simulink model "Switch"  (R2017b)
settings: Solver=FixedStepAuto  StartTime=0.0  StopTime=10.0  FixedStep=0.1  RelTol=1e-3  EnableMultiTasking=on
settings Model: Creator=ktrinh  LastModifiedBy=hbourbou
settings DataIOCC: SaveFormat=StructureWithTime
settings OptimizationCC: LifeSpan=inf
settings DebuggingCC: SFUnexpectedBacktrackingDiag=warning  SFNoUnconditionalDefaultTransitionDiag=warning  SFExecutionAtInitializationDiag=none
settings HardwareCC: ProdBitPerSizeT=32  ProdBitPerPtrDiffT=32  ProdWordSize=32  ProdHWDeviceType=Specified
settings CodeAppCC: StateflowObjectComments=on
settings GRTTargetCC: TargetLangStandard=C89/C90 (ANSI)  GeneratePreprocessorConditionals=Disable all
settings ConfigComp: CovMetricSettings=dw  CovHtmlReporting=on  CovSaveCumulativeToWorkspaceVar=on  CovSaveSingleToWorkspaceVar=on  CovExternalEMLEnable=off

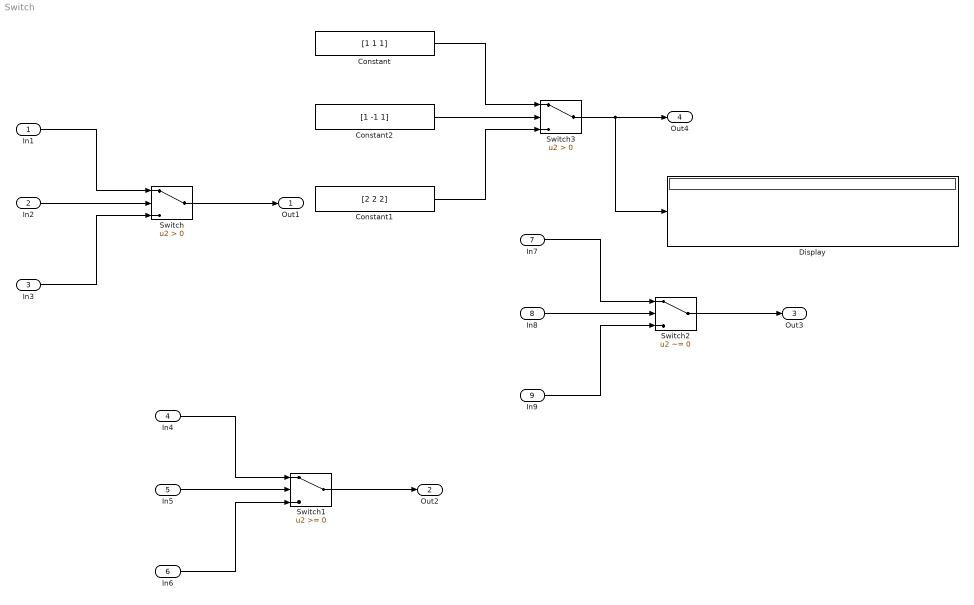
== system Switch ==
  In1 : Inport  OutMin=5  OutDataTypeStr=uint8  PortDimensions=3
  In2 : Inport  Port=2  PortDimensions=3
  In3 : Inport  Port=3  PortDimensions=3
  In4 : Inport  Port=4
  In5 : Inport  Port=5
  In6 : Inport  Port=6
  In7 : Inport  Port=7
  In8 : Inport  Port=8
  In9 : Inport  Port=9
  Constant : Constant  Value=[1 1 1]
  Constant1 : Constant  Value=[2 2 2]
  Constant2 : Constant  Value=[1 -1 1]
  Display : Display
  Switch : Switch  Criteria=u2 > Threshold
  Switch1 : Switch
  Switch2 : Switch  Criteria=u2 ~= 0
  Switch3 : Switch  Criteria=u2 > Threshold
  Out1 : Outport
  Out2 : Outport  Port=2
  Out3 : Outport  Port=3
  Out4 : Outport  Port=4
  wires:
  Switch/1 -> Out1/1
  In1/1 -> Switch/1
  In2/1 -> Switch/2
  In3/1 -> Switch/3
  Switch1/1 -> Out2/1
  In4/1 -> Switch1/1
  In5/1 -> Switch1/2
  In6/1 -> Switch1/3
  Switch2/1 -> Out3/1
  In7/1 -> Switch2/1
  In8/1 -> Switch2/2
  In9/1 -> Switch2/3
  Switch3/1 -> Display/1, Out4/1
  Constant/1 -> Switch3/1
  Constant2/1 -> Switch3/2
  Constant1/1 -> Switch3/3
